simulink model "lab7_model"  (R2023a)
settings: Solver=VariableStepAuto  StartTime=0.0  StopTime=15  FixedStep=0.001  RelTol=1e-3
values from neighbouring files (symbols this model uses):
  alpha = Rr/Lr    (= 3.74100719424)    [Laboratory7.m]    (also in lab7.m)
  beta = LM/gamma/Ls/Lr    (= 470.831419384)    [Laboratory7.m]    (also in lab7.m)
  f = 50    [Laboratory7.m]    (also in lab7.m)
  gamma = 1 - LM^2/Ls/Lr    (= 0.0492511651057)    [Laboratory7.m]    (also in lab7.m)
  J = 0.4    [Laboratory7.m]    (also in lab7.m)
  Kf = 0.1115    [Laboratory7.m]    (also in lab7.m)
  Kr_PI = 0.45 * K0    (= 15.7406020421)    [Laboratory7.m]    (also in lab7.m)
  LM = 0.041    [Laboratory7.m]    (also in lab7.m)
  Lr = 0.0417    [Laboratory7.m]    (also in lab7.m)
  Ls = 0.0424    [Laboratory7.m]    (also in lab7.m)
  MR = 0    [Laboratory7.m]    (also in lab7.m)
  Rs = 0.294    [Laboratory7.m]    (also in lab7.m)
  Ti_PI = 0.8 * T0    (= 5.6536)    [Laboratory7.m]    (also in lab7.m)
libraries: slpidlib x2, commsynccomp2 x2
settings Model: Creator=evely  LastModifiedBy=evely

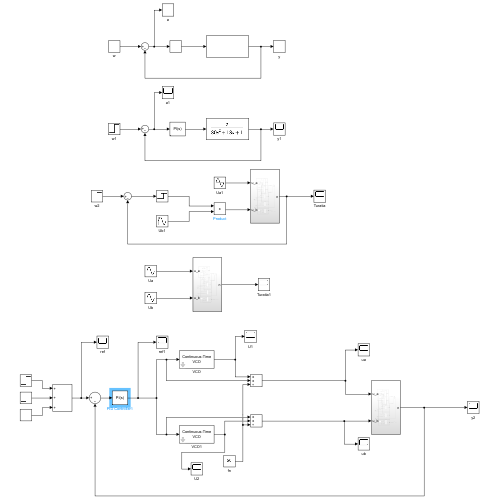
[thumbnail: Simulink's stored preview of the top-level diagram]
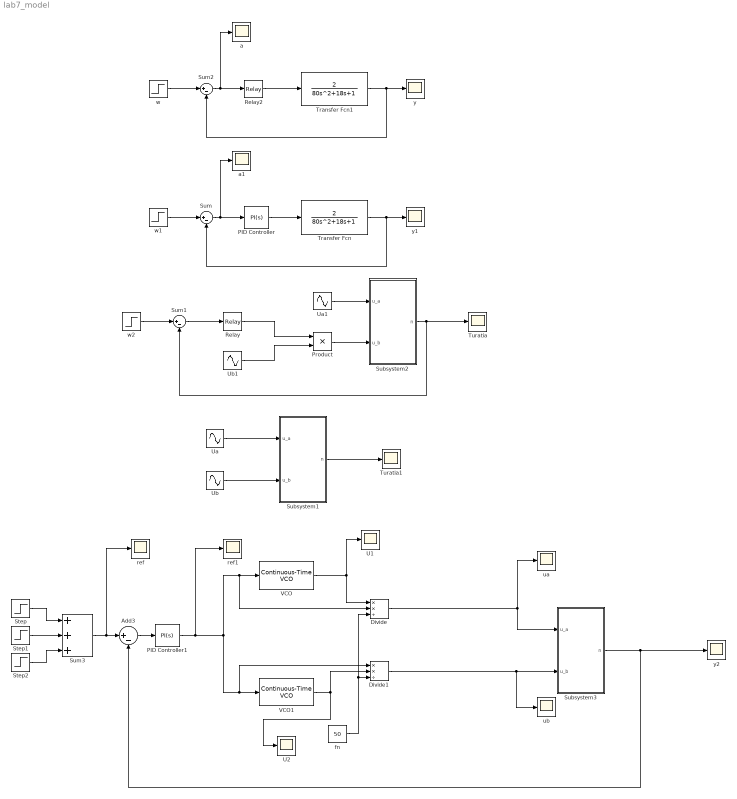
== system lab7_model ==
  Add3 : Sum  Inputs=|+-
  Divide : Product  Inputs=**/
  Divide1 : Product  Inputs=**/
  PID Controller : slpidlib/PID Controller  Controller=PI  Form=Ideal  TimeDomain=Continuous-time  UseExternalTs=off  SampleTime=-1  IntegratorMethod=Forward Euler  FilterMethod=Forward Euler  ControllerParametersSource=internal  P=Kr_PI  I=1/Ti_PI  UseKiTs=off  D=0  N=100  UseFilter=on  TunerSelectOption=Transfer Function Based (PID Tuner App)  InitialConditionSource=internal  InitialConditionForIntegrator=0  InitialConditionForFilter=0  DifferentiatorICPrevScaledInput=0  ExternalReset=none  TrackingMode=off  Kt=1  LimitOutput=off  SatLimitsSource=internal  UpperSaturationLimit=inf  LowerSaturationLimit=-inf  LinearizeAsGain=on  AntiWindupMode=none  Kb=1  LimitIntegrator=off  UpperIntegratorSaturationLimit=inf  LowerIntegratorSaturationLimit=-inf  POutMin=[]  POutMax=[]  IOutMin=[]  IOutMax=[]  DOutMin=[]  DOutMax=[]  NOutMin=[]  NOutMax=[]  SumOutMin=[]  SumOutMax=[]  SaturationOutMin=[]  SaturationOutMax=[]  PParamMin=[]  PParamMax=[]  IParamMin=[]  IParamMax=[]  DParamMin=[]  DParamMax=[]  NParamMin=[]  NParamMax=[]  KbParamMin=[]  KbParamMax=[]  KtParamMin=[]  KtParamMax=[]  KbOutMin=[]  KbOutMax=[]  KtOutMin=[]  KtOutMax=[]  IntegratorOutMin=[]  IntegratorOutMax=[]  FilterOutMin=[]  FilterOutMax=[]  SumI1OutMin=[]  SumI1OutMax=[]  SumI2OutMin=[]  SumI2OutMax=[]  SumI3OutMin=[]  SumI3OutMax=[]  SumI4OutMin=[]  SumI4OutMax=[]  SumDOutMin=[]  SumDOutMax=[]  DifferentiatorOutMin=[]  DifferentiatorOutMax=[]  FilterDiffOutCoefMin=[]  FilterDiffOutCoefMax=[]  ReciprocalOutMin=[]  ReciprocalOutMax=[]  SumDenOutMin=[]  SumDenOutMax=[]  SumNumOutMin=[]  SumNumOutMax=[]  DivideOutMin=[]  DivideOutMax=[]  UdiffTsProdOutMin=[]  UdiffTsProdOutMax=[]  NTsProdOutMin=[]  NTsProdOutMax=[]  UintegralTsProdOutMin=[]  UintegralTsProdOutMax=[]  UngainTsProdOutMin=[]  UngainTsProdOutMax=[]  ClampingZeroOutDataTypeStr=Inherit: Inherit via back propagation  ClampingZeroOutMin=[]  ClampingZeroOutMax=[]  FilterDenConstantOutDataTypeStr=Inherit: Inherit via back propagation  FilterDenConstantOutMin=[]  FilterDenConstantOutMax=[]  PCopyOutDataTypeStr=Inherit: Inherit via back propagation  PCopyOutMin=[]  PCopyOutMax=[]  NCopyOutDataTypeStr=Inherit: Inherit via back propagation  NCopyOutMin=[]  NCopyOutMax=[]  IntegratorContinuousStateAttributes=''  IntegratorStateMustResolveToSignalObject=off  IntegratorRTWStateStorageClass=Auto  FilterContinuousStateAttributes=''  FilterStateMustResolveToSignalObject=off  FilterRTWStateStorageClass=Auto  ParallelPVariant=Passthrough  IdealPVariant=InternalParameters  IVariant=InternalParameters  DVariant=Disabled  IntegratorVariant=Continuous  SatVariant=Disabled  AWVariant=Passthrough  PCopyVariant=Disabled  TRVariant=Disabled  FdbkBlocksVariant=Forward  IdealPFdbkVariant=Disabled  SatFdbkVariant=Disabled  DerivativeFilterVariant=Disabled  NVariant=Disabled  NCopyVariant=Disabled_SignalSpec  FilterICVariant=Disabled  IntegratorICVariant=InternalICs  ExternalResetVariant=Disabled  TRSumVariant=Passthrough  SumFdbkVariant=Disabled  SumVariant=Sum_PI  TsampFilterVariant=InternalTs  TsampNgainVariant=Passthrough  TsampIntegralVariant=Disabled_SignalSpec  ExternalSaturationOutDataTypeStr=Inherit: Same as second input
  PID Controller1 : slpidlib/PID Controller  Controller=PI  Form=Ideal  TimeDomain=Continuous-time  UseExternalTs=off  SampleTime=-1  IntegratorMethod=Forward Euler  FilterMethod=Forward Euler  ControllerParametersSource=internal  P=0.0027  I=1/0.096  UseKiTs=off  D=0  N=100  UseFilter=on  TunerSelectOption=Transfer Function Based (PID Tuner App)  InitialConditionSource=internal  InitialConditionForIntegrator=0  InitialConditionForFilter=0  DifferentiatorICPrevScaledInput=0  ExternalReset=none  TrackingMode=off  Kt=1  LimitOutput=off  SatLimitsSource=internal  UpperSaturationLimit=inf  LowerSaturationLimit=-inf  LinearizeAsGain=on  AntiWindupMode=none  Kb=1  LimitIntegrator=off  UpperIntegratorSaturationLimit=inf  LowerIntegratorSaturationLimit=-inf  POutMin=[]  POutMax=[]  IOutMin=[]  IOutMax=[]  DOutMin=[]  DOutMax=[]  NOutMin=[]  NOutMax=[]  SumOutMin=[]  SumOutMax=[]  SaturationOutMin=[]  SaturationOutMax=[]  PParamMin=[]  PParamMax=[]  IParamMin=[]  IParamMax=[]  DParamMin=[]  DParamMax=[]  NParamMin=[]  NParamMax=[]  KbParamMin=[]  KbParamMax=[]  KtParamMin=[]  KtParamMax=[]  KbOutMin=[]  KbOutMax=[]  KtOutMin=[]  KtOutMax=[]  IntegratorOutMin=[]  IntegratorOutMax=[]  FilterOutMin=[]  FilterOutMax=[]  SumI1OutMin=[]  SumI1OutMax=[]  SumI2OutMin=[]  SumI2OutMax=[]  SumI3OutMin=[]  SumI3OutMax=[]  SumI4OutMin=[]  SumI4OutMax=[]  SumDOutMin=[]  SumDOutMax=[]  DifferentiatorOutMin=[]  DifferentiatorOutMax=[]  FilterDiffOutCoefMin=[]  FilterDiffOutCoefMax=[]  ReciprocalOutMin=[]  ReciprocalOutMax=[]  SumDenOutMin=[]  SumDenOutMax=[]  SumNumOutMin=[]  SumNumOutMax=[]  DivideOutMin=[]  DivideOutMax=[]  UdiffTsProdOutMin=[]  UdiffTsProdOutMax=[]  NTsProdOutMin=[]  NTsProdOutMax=[]  UintegralTsProdOutMin=[]  UintegralTsProdOutMax=[]  UngainTsProdOutMin=[]  UngainTsProdOutMax=[]  ClampingZeroOutDataTypeStr=Inherit: Inherit via back propagation  ClampingZeroOutMin=[]  ClampingZeroOutMax=[]  FilterDenConstantOutDataTypeStr=Inherit: Inherit via back propagation  FilterDenConstantOutMin=[]  FilterDenConstantOutMax=[]  PCopyOutDataTypeStr=Inherit: Inherit via back propagation  PCopyOutMin=[]  PCopyOutMax=[]  NCopyOutDataTypeStr=Inherit: Inherit via back propagation  NCopyOutMin=[]  NCopyOutMax=[]  IntegratorContinuousStateAttributes=''  IntegratorStateMustResolveToSignalObject=off  IntegratorRTWStateStorageClass=Auto  FilterContinuousStateAttributes=''  FilterStateMustResolveToSignalObject=off  FilterRTWStateStorageClass=Auto  ParallelPVariant=Passthrough  IdealPVariant=InternalParameters  IVariant=InternalParameters  DVariant=Disabled  IntegratorVariant=Continuous  SatVariant=Disabled  AWVariant=Passthrough  PCopyVariant=Disabled  TRVariant=Disabled  FdbkBlocksVariant=Forward  IdealPFdbkVariant=Disabled  SatFdbkVariant=Disabled  DerivativeFilterVariant=Disabled  NVariant=Disabled  NCopyVariant=Disabled_SignalSpec  FilterICVariant=Disabled  IntegratorICVariant=InternalICs  ExternalResetVariant=Disabled  TRSumVariant=Passthrough  SumFdbkVariant=Disabled  SumVariant=Sum_PI  TsampFilterVariant=InternalTs  TsampNgainVariant=Passthrough  TsampIntegralVariant=Disabled_SignalSpec  ExternalSaturationOutDataTypeStr=Inherit: Same as second input
  Product : Product
  Relay : Relay  OnSwitchValue=0.01  OffSwitchValue=-0.01  OffOutputValue=-1
  Relay2 : Relay  OnSwitchValue=0.01  OffSwitchValue=-0.01  OffOutputValue=-1
  Step : Step  Time=0  After=1000  SampleTime=0
  Step1 : Step  Time=5  After=1000  SampleTime=0
  Step2 : Step  Time=10  After=-500  SampleTime=0
  Subsystem1 : Subsystem
  Subsystem2 : Subsystem
  Subsystem3 : Subsystem
  Sum : Sum  Inputs=|+-
  Sum1 : Sum  Inputs=|+-
  Sum2 : Sum  Inputs=|+-
  Sum3 : Sum  Inputs=+++
  Transfer Fcn : TransferFcn  Numerator=2  Denominator=[80, 18, 1]
  Transfer Fcn1 : TransferFcn  Numerator=2  Denominator=[80, 18, 1]
  Turatia : Scope
  Turatia1 : Scope
  U1 : Scope
  U2 : Scope
  Ua : Sin  Amplitude=220*sqrt(2)  Frequency=2*pi*f  Phase=pi/2  SampleTime=0
  Ua1 : Sin  Amplitude=220*sqrt(2)  Frequency=2*pi*f  Phase=pi/2  SampleTime=0
  Ub : Sin  Amplitude=220*sqrt(2)  Frequency=2*pi*f  SampleTime=0
  Ub1 : Sin  Amplitude=220*sqrt(2)  Frequency=2*pi*f  SampleTime=0
  VCO : commsynccomp2/Continuous-Time VCO  Ac=220*sqrt(2)  Fc=0  Kc=1  Ph=pi/2
  VCO1 : commsynccomp2/Continuous-Time VCO  Ac=220*sqrt(2)  Fc=0  Kc=1  Ph=0
  a : Scope
  a1 : Scope
  fn : Constant  Value=50
  ref : Scope
  ref1 : Scope
  ua : Scope
  ub : Scope
  w : Step  After=0  SampleTime=0
  w1 : Step  SampleTime=0
  w2 : Step  Before=f  After=f  SampleTime=0
  y : Scope
  y1 : Scope
  y2 : Scope
  wires:
  Transfer Fcn/1 -> Sum/2, y1/1
  Sum/1 -> PID Controller/1, a1/1
  w1/1 -> Sum/1
  Relay2/1 -> Transfer Fcn1/1
  w/1 -> Sum2/1
  Transfer Fcn1/1 -> Sum2/2, y/1
  Sum2/1 -> a/1, Relay2/1
  PID Controller/1 -> Transfer Fcn/1
  w2/1 -> Sum1/1
  Sum1/1 -> Relay/1
  Subsystem2/1(n) -> Sum1/2, Turatia/1
  Ua1/1 -> Subsystem2/1(u_a)
  Product/1 -> Subsystem2/2(u_b)
  Ub1/1 -> Product/2
  Relay/1 -> Product/1
  Step2/1 -> Sum3/3
  fn/1 -> Divide/3, Divide1/3
  PID Controller1/1 -> ref1/1, VCO/1, Divide/2, Divide1/1, VCO1/1
  Step1/1 -> Sum3/2
  Subsystem3/1(n) -> y2/1, Add3/2
  Divide1/1 -> Subsystem3/2(u_b), ub/1
  VCO/1 -> U1/1, Divide/1
  Divide/1 -> Subsystem3/1(u_a), ua/1
  Sum3/1 -> ref/1, Add3/1
  VCO1/1 -> U2/1, Divide1/2
  Step/1 -> Sum3/1
  Add3/1 -> PID Controller1/1
  Subsystem1/1(n) -> Turatia1/1
  Ub/1 -> Subsystem1/2(u_b)
  Ua/1 -> Subsystem1/1(u_a)

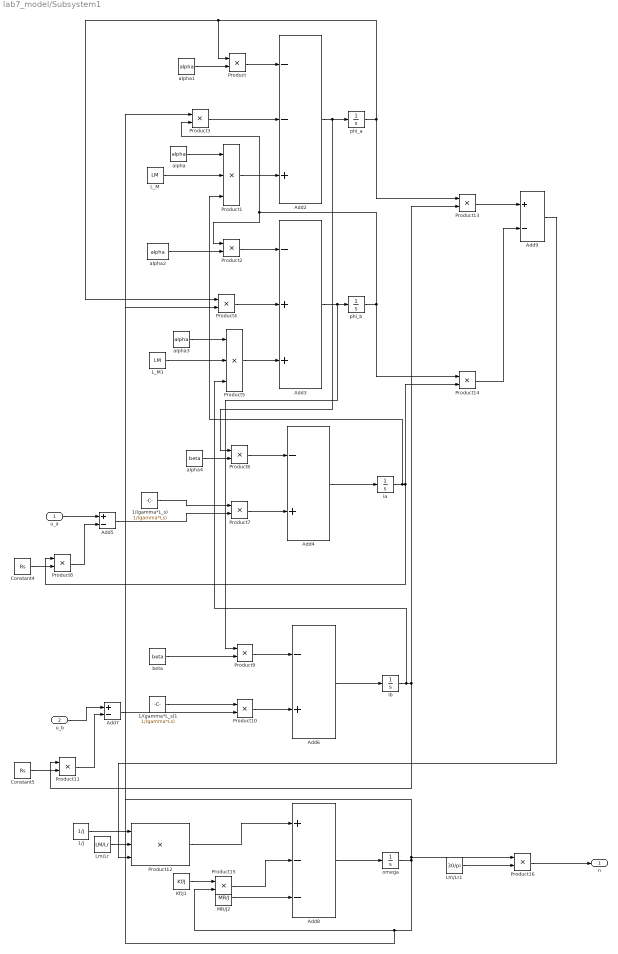
== system lab7_model/Subsystem1 ==
  u_a : Inport
  u_b : Inport  Port=2
  1/(gamma*L_s) : Constant  Value=1/(gamma*Ls)
  1/(gamma*L_s)1 : Constant  Value=1/(gamma*Ls)
  1/J : Constant  Value=1/J
  Add2 : Sum  Inputs=--+
  Add3 : Sum  Inputs=-++
  Add4 : Sum  Inputs=-+
  Add5 : Sum  Inputs=+-
  Add6 : Sum  Inputs=-+
  Add7 : Sum  Inputs=+-
  Add8 : Sum  Inputs=+--
  Add9 : Sum  Inputs=+-
  Constant4 : Constant  Value=Rs
  Constant5 : Constant  Value=Rs
  Kf/J1 : Constant  Value=Kf/J
  L_M : Constant  Value=LM
  L_M1 : Constant  Value=LM
  Lm/Lr : Constant  Value=LM/Lr
  Lm/Lr1 : Constant  Value=30/pi
  MR/J2 : Constant  Value=MR/J
  Product{,2..4,6..11,13..16} (14 alike) : Product
  Product1 : Product  Inputs=3
  Product12 : Product  Inputs=3
  Product5 : Product  Inputs=3
  alpha{,1..3} (4 alike) : Constant  Value=alpha
  alpha4 : Constant  Value=beta
  beta : Constant  Value=beta
  ia : Integrator
  ib : Integrator
  omega : Integrator
  phi_a : Integrator
  phi_b : Integrator
  n : Outport
  wires:
  Lm/Lr1/1 -> Product16/2
  L_M1/1 -> Product5/2
  Product8/1 -> Add5/2
  Product/1 -> Add2/1
  u_b/1 -> Add7/1
  Product16/1 -> n/1
  Add8/1 -> omega/1
  phi_a/1 -> Product4/1, Product/1, Product13/1
  Add2/1 -> Product6/1, phi_a/1
  1/(gamma*L_s)/1 -> Product7/1
  Product5/1 -> Add3/3
  Product4/1 -> Add3/2
  Product15/1 -> Add8/2
  1/J/1 -> Product12/1
  Product13/1 -> Add9/1
  Product3/1 -> Add2/2
  MR/J2/1 -> Add8/3
  phi_b/1 -> Product3/2, Product2/1, Product14/1
  Product14/1 -> Add9/2
  Kf/J1/1 -> Product15/1
  Add5/1 -> Product7/2
  alpha2/1 -> Product2/2
  Product11/1 -> Add7/2
  Add4/1 -> ia/1
  u_a/1 -> Add5/1
  Product6/1 -> Add4/1
  ib/1 -> Product11/1, Product13/2, Product5/3
  Lm/Lr/1 -> Product12/2
  alpha/1 -> Product1/1
  Product12/1 -> Add8/1
  Product9/1 -> Add6/1
  L_M/1 -> Product1/2
  Constant5/1 -> Product11/2
  ia/1 -> Product1/3, Product8/1, Product14/2
  Add7/1 -> Product10/2
  alpha1/1 -> Product/2
  Add9/1 -> Product12/3
  Product2/1 -> Add3/1
  Product10/1 -> Add6/2
  Product7/1 -> Add4/2
  Add6/1 -> ib/1
  1/(gamma*L_s)1/1 -> Product10/1
  Constant4/1 -> Product8/2
  Product1/1 -> Add2/3
  beta/1 -> Product9/2
  Add3/1 -> Product9/1, phi_b/1
  alpha3/1 -> Product5/1
  omega/1 -> Product16/1, Product3/1, Product4/2, Product15/2
  alpha4/1 -> Product6/2

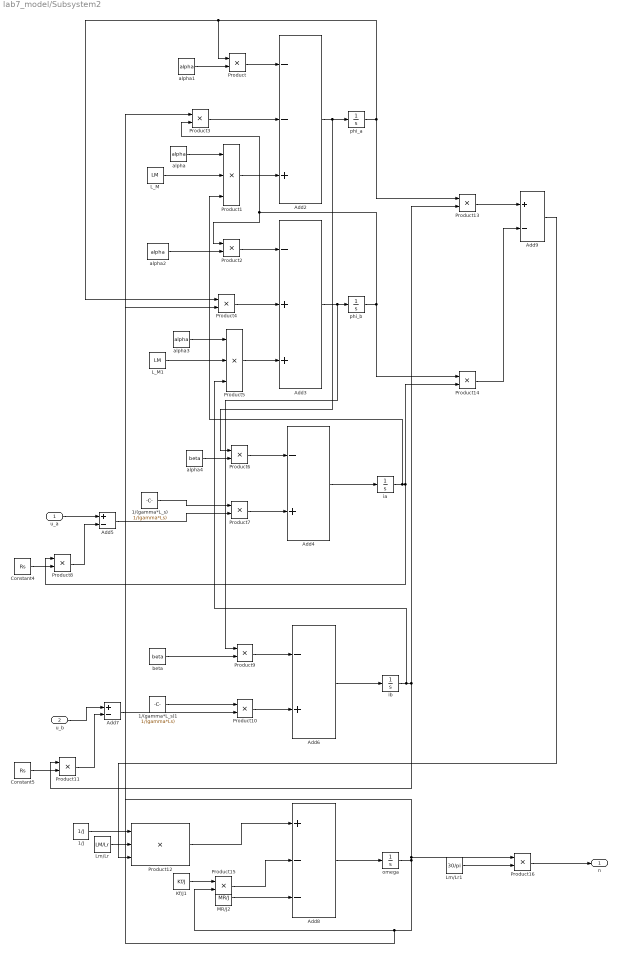
== system lab7_model/Subsystem2 ==
  u_a : Inport
  u_b : Inport  Port=2
  1/(gamma*L_s) : Constant  Value=1/(gamma*Ls)
  1/(gamma*L_s)1 : Constant  Value=1/(gamma*Ls)
  1/J : Constant  Value=1/J
  Add2 : Sum  Inputs=--+
  Add3 : Sum  Inputs=-++
  Add4 : Sum  Inputs=-+
  Add5 : Sum  Inputs=+-
  Add6 : Sum  Inputs=-+
  Add7 : Sum  Inputs=+-
  Add8 : Sum  Inputs=+--
  Add9 : Sum  Inputs=+-
  Constant4 : Constant  Value=Rs
  Constant5 : Constant  Value=Rs
  Kf/J1 : Constant  Value=Kf/J
  L_M : Constant  Value=LM
  L_M1 : Constant  Value=LM
  Lm/Lr : Constant  Value=LM/Lr
  Lm/Lr1 : Constant  Value=30/pi
  MR/J2 : Constant  Value=MR/J
  Product{,2..4,6..11,13..16} (14 alike) : Product
  Product1 : Product  Inputs=3
  Product12 : Product  Inputs=3
  Product5 : Product  Inputs=3
  alpha{,1..3} (4 alike) : Constant  Value=alpha
  alpha4 : Constant  Value=beta
  beta : Constant  Value=beta
  ia : Integrator
  ib : Integrator
  omega : Integrator
  phi_a : Integrator
  phi_b : Integrator
  n : Outport
  wires:
  Lm/Lr1/1 -> Product16/2
  L_M1/1 -> Product5/2
  Product8/1 -> Add5/2
  Product/1 -> Add2/1
  u_b/1 -> Add7/1
  Product16/1 -> n/1
  Add8/1 -> omega/1
  phi_a/1 -> Product4/1, Product/1, Product13/1
  Add2/1 -> Product6/1, phi_a/1
  1/(gamma*L_s)/1 -> Product7/1
  Product5/1 -> Add3/3
  Product4/1 -> Add3/2
  Product15/1 -> Add8/2
  1/J/1 -> Product12/1
  Product13/1 -> Add9/1
  Product3/1 -> Add2/2
  MR/J2/1 -> Add8/3
  phi_b/1 -> Product3/2, Product2/1, Product14/1
  Product14/1 -> Add9/2
  Kf/J1/1 -> Product15/1
  Add5/1 -> Product7/2
  alpha2/1 -> Product2/2
  Product11/1 -> Add7/2
  Add4/1 -> ia/1
  u_a/1 -> Add5/1
  Product6/1 -> Add4/1
  ib/1 -> Product11/1, Product13/2, Product5/3
  Lm/Lr/1 -> Product12/2
  alpha/1 -> Product1/1
  Product12/1 -> Add8/1
  Product9/1 -> Add6/1
  L_M/1 -> Product1/2
  Constant5/1 -> Product11/2
  ia/1 -> Product1/3, Product8/1, Product14/2
  Add7/1 -> Product10/2
  alpha1/1 -> Product/2
  Add9/1 -> Product12/3
  Product2/1 -> Add3/1
  Product10/1 -> Add6/2
  Product7/1 -> Add4/2
  Add6/1 -> ib/1
  1/(gamma*L_s)1/1 -> Product10/1
  Constant4/1 -> Product8/2
  Product1/1 -> Add2/3
  beta/1 -> Product9/2
  Add3/1 -> Product9/1, phi_b/1
  alpha3/1 -> Product5/1
  omega/1 -> Product16/1, Product3/1, Product4/2, Product15/2
  alpha4/1 -> Product6/2

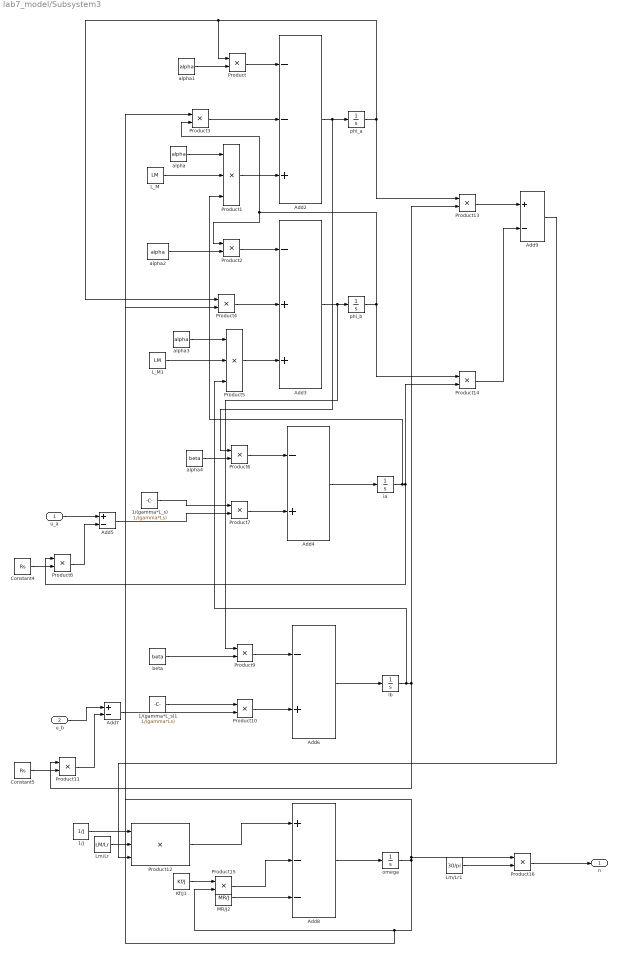
== system lab7_model/Subsystem3 ==
  u_a : Inport
  u_b : Inport  Port=2
  1/(gamma*L_s) : Constant  Value=1/(gamma*Ls)
  1/(gamma*L_s)1 : Constant  Value=1/(gamma*Ls)
  1/J : Constant  Value=1/J
  Add2 : Sum  Inputs=--+
  Add3 : Sum  Inputs=-++
  Add4 : Sum  Inputs=-+
  Add5 : Sum  Inputs=+-
  Add6 : Sum  Inputs=-+
  Add7 : Sum  Inputs=+-
  Add8 : Sum  Inputs=+--
  Add9 : Sum  Inputs=+-
  Constant4 : Constant  Value=Rs
  Constant5 : Constant  Value=Rs
  Kf/J1 : Constant  Value=Kf/J
  L_M : Constant  Value=LM
  L_M1 : Constant  Value=LM
  Lm/Lr : Constant  Value=LM/Lr
  Lm/Lr1 : Constant  Value=30/pi
  MR/J2 : Constant  Value=MR/J
  Product{,2..4,6..11,13..16} (14 alike) : Product
  Product1 : Product  Inputs=3
  Product12 : Product  Inputs=3
  Product5 : Product  Inputs=3
  alpha{,1..3} (4 alike) : Constant  Value=alpha
  alpha4 : Constant  Value=beta
  beta : Constant  Value=beta
  ia : Integrator
  ib : Integrator
  omega : Integrator
  phi_a : Integrator
  phi_b : Integrator
  n : Outport
  wires:
  Lm/Lr1/1 -> Product16/2
  L_M1/1 -> Product5/2
  Product8/1 -> Add5/2
  Product/1 -> Add2/1
  u_b/1 -> Add7/1
  Product16/1 -> n/1
  Add8/1 -> omega/1
  phi_a/1 -> Product4/1, Product/1, Product13/1
  Add2/1 -> Product6/1, phi_a/1
  1/(gamma*L_s)/1 -> Product7/1
  Product5/1 -> Add3/3
  Product4/1 -> Add3/2
  Product15/1 -> Add8/2
  1/J/1 -> Product12/1
  Product13/1 -> Add9/1
  Product3/1 -> Add2/2
  MR/J2/1 -> Add8/3
  phi_b/1 -> Product3/2, Product2/1, Product14/1
  Product14/1 -> Add9/2
  Kf/J1/1 -> Product15/1
  Add5/1 -> Product7/2
  alpha2/1 -> Product2/2
  Product11/1 -> Add7/2
  Add4/1 -> ia/1
  u_a/1 -> Add5/1
  Product6/1 -> Add4/1
  ib/1 -> Product11/1, Product13/2, Product5/3
  Lm/Lr/1 -> Product12/2
  alpha/1 -> Product1/1
  Product12/1 -> Add8/1
  Product9/1 -> Add6/1
  L_M/1 -> Product1/2
  Constant5/1 -> Product11/2
  ia/1 -> Product1/3, Product8/1, Product14/2
  Add7/1 -> Product10/2
  alpha1/1 -> Product/2
  Add9/1 -> Product12/3
  Product2/1 -> Add3/1
  Product10/1 -> Add6/2
  Product7/1 -> Add4/2
  Add6/1 -> ib/1
  1/(gamma*L_s)1/1 -> Product10/1
  Constant4/1 -> Product8/2
  Product1/1 -> Add2/3
  beta/1 -> Product9/2
  Add3/1 -> Product9/1, phi_b/1
  alpha3/1 -> Product5/1
  omega/1 -> Product16/1, Product3/1, Product4/2, Product15/2
  alpha4/1 -> Product6/2
